simulink model "Blinker_31_exp_func_call_final"  (R2020b)
settings: Solver=FixedStepDiscrete  StartTime=0.0  StopTime=10.0  FixedStep=Ts  RelTol=1e-3  EnableMultiTasking=on
PreLoadFcn:
  | Ts = 0.05;
  | Ts_1 = 0.05;   % for runnable blink_signal
  | Ts_2 = 1;       % for runnable validate_ignition
  | 
  | SetEnumTypeBlink;
undefined symbols (not defined in the file or in its folder): BlinkerValues
libraries: simulink x1
settings Model: SimSIMDOptimization=Portable  Creator=urempel  LastModifiedBy=bnewman
settings DataIOCC: LimitDataPoints=on  SaveFormat=Array  ReturnWorkspaceOutputs=off
settings OptimizationCC: ZeroExternalMemoryAtStartup=off  ZeroInternalMemoryAtStartup=off  LifeSpan=1  EfficientTunableParamExpr=on
settings DebuggingCC: SolverPrmCheckMsg=warning  AllowSymbolicDim=off  SFUnexpectedBacktrackingDiag=warning  SFNoUnconditionalDefaultTransitionDiag=warning  SFExecutionAtInitializationDiag=none  ArithmeticOperatorsInVariantConditions=warning
settings ModelReferenceCC: ModelReferenceNumInstancesAllowed=Single  PropagateSignalLabelsOutOfModel=off
settings SFSimCC: SimUseLocalCustomCode=off  SimGenImportedTypeDefs=on  MATLABDynamicMemAlloc=off  CustomCodeUndefinedFunction=UseInterfaceOnly
settings RTWCC: Description=AUTOSAR  SystemTargetFile=autosar.tlc  GenCodeOnly=on  TemplateMakefile=ert_default_tmf  RTWUseLocalCustomCode=off  IncludeHyperlinkInReport=on  GenerateCodeMetricsReport=on
settings CodeAppCC: IgnoreCustomStorageClasses=off  StateflowObjectComments=on
settings STFCustomTargetCC: ParMdlRefBuildCompliant=on  CompOptLevelCompliant=on  ConcurrentExecutionCompliant=off  IncludeMdlTerminateFcn=off  CombineOutputUpdateFcns=on  SuppressErrorStatus=on  ERTCustomFileBanners=on  SupportNonFinite=off  SupportComplex=off  SupportContinuousTime=off  SupportNonInlinedSFcns=off  RemoveResetFunc=on  MATLABClassNameForMDSCustomization=Simulink.SoftwareTarget.ERTCustomization  CPPClassGenCompliant=off  AutosarCompliant=on  GRTInterface=off  UseToolchainInfoCompliant=on  LookupTableObjectStructAxisOrder=2,1,3,4,...  LUTObjectStructOrderEvenSpacing=Size,Table,Breakpoints  SystemTargetFile=autosar.tlc
settings ERTTargetCC: MultiwordLength=2048  ConcurrentExecutionCompliant=off  IncludeMdlTerminateFcn=off  SuppressErrorStatus=on  SupportNonFinite=off  SupportComplex=off  ModelStepFunctionPrototypeControlCompliant=off  CPPClassGenCompliant=off  AutosarCompliant=on  LookupTableObjectStructAxisOrder=2,1,3,4,...  LUTObjectStructOrderEvenSpacing=Size,Table,Breakpoints  ERTCustomFileTemplate=example_file_process.tlc  ERTFilePackagingFormat=CompactWithDataFile  ConvertIfToSwitch=off  SuppressUnreachableDefaultCases=off
settings ConfigComp: CovMetricSettings=dw  CovSaveCumulativeToWorkspaceVar=on  CovSaveSingleToWorkspaceVar=on  CovExternalEMLEnable=off  CovSFcnEnable=off

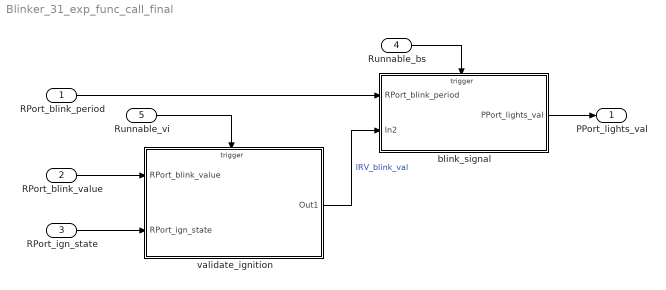
== system Blinker_31_exp_func_call_final ==
  RPort_blink_period : Inport  OutDataTypeStr=uint32
      settings: AttributesFormatString=%<OutDataTypeStr>
  RPort_blink_value : Inport  Port=2  OutDataTypeStr=Enum: BlinkerValues
      settings: AttributesFormatString=%<OutDataTypeStr>
  RPort_ign_state : Inport  Port=3  OutDataTypeStr=boolean
      settings: AttributesFormatString=%<OutDataTypeStr>
  Runnable_bs : Inport  Port=4  SampleTime=Ts_1  OutputFunctionCall=on
  Runnable_vi : Inport  Port=5  SampleTime=Ts_2  OutputFunctionCall=on
  blink_signal : Subsystem
  validate_ignition : Subsystem
  PPort_lights_val : Outport  InitialOutput=0  VectorParamsAs1DForOutWhenUnconnected=off
  wires:
  RPort_blink_value/1 -> validate_ignition/1(RPort_blink_value)
  RPort_ign_state/1 -> validate_ignition/2(RPort_ign_state)
  RPort_blink_period/1 -> blink_signal/1(RPort_blink_period)
  validate_ignition/1(Out1) -> blink_signal/2(In2)  "IRV_blink_val"
  blink_signal/1(PPort_lights_val) -> PPort_lights_val/1
  Runnable_bs/1 -> blink_signal/Trigger
  Runnable_vi/1 -> validate_ignition/Trigger

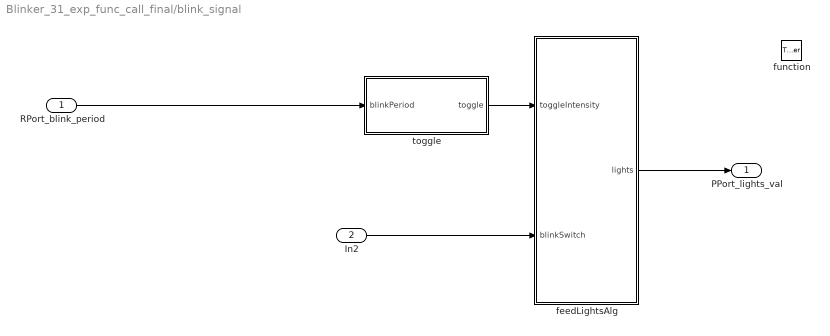
== system Blinker_31_exp_func_call_final/blink_signal ==
  RPort_blink_period : Inport  OutDataTypeStr=uint32
      settings: AttributesFormatString=%<OutDataTypeStr>
  In2 : Inport  Port=2
  function : TriggerPort  TriggerType=function-call  VariantControl=(inherit)  SampleTimeType=periodic  SampleTime=-1
  feedLightsAlg : MATLAB Function  TreatAsAtomicUnit=on
  toggle : Stateflow chart  TreatAsAtomicUnit=on
  PPort_lights_val : Outport  InitialOutput=0  VectorParamsAs1DForOutWhenUnconnected=off
  wires:
  RPort_blink_period/1 -> toggle/1(blinkPeriod)
  feedLightsAlg/1(lights) -> PPort_lights_val/1
  toggle/1(toggle) -> feedLightsAlg/1(toggleIntensity)
  In2/1 -> feedLightsAlg/2(blinkSwitch)

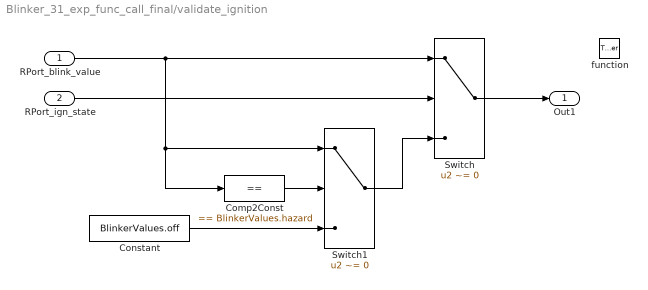
== system Blinker_31_exp_func_call_final/validate_ignition ==
  RPort_blink_value : Inport  OutDataTypeStr=Enum: BlinkerValues
      settings: AttributesFormatString=%<OutDataTypeStr>
  RPort_ign_state : Inport  Port=2  OutDataTypeStr=boolean
      settings: AttributesFormatString=%<OutDataTypeStr>
  function : TriggerPort  TriggerType=function-call  VariantControl=(inherit)  SampleTimeType=periodic  SampleTime=-1
  Comp2Const : simulink/Logic and Bit Operations/Compare To Constant  relop===  const=BlinkerValues.hazard  OutDataTypeStr=boolean
  Constant : Constant  Value=BlinkerValues.off
      settings: AttributesFormatString=%<OutDataTypeStr>
  Switch : Switch  Criteria=u2 ~= 0
  Switch1 : Switch  Criteria=u2 ~= 0
  Out1 : Outport  VectorParamsAs1DForOutWhenUnconnected=off
  wires:
  Switch1/1 -> Switch/3
  RPort_blink_value/1 -> Switch1/1, Comp2Const/1, Switch/1
  Comp2Const/1 -> Switch1/2
  RPort_ign_state/1 -> Switch/2
  Switch/1 -> Out1/1
  Constant/1 -> Switch1/3

== matlab function Blinker_31_exp_func_call_final/blink_signal/feedLightsAlg ==
  data: toggleIntensity input boolean; blinkSwitch input Enum: BlinkerValues; lights output boolean size=[1,2]
function lights = feedLightsAlg(toggleIntensity, blinkSwitch )
%#codegen
switch blinkSwitch
	case BlinkerValues.right
		lights = [false, toggleIntensity];
	case BlinkerValues.left
		lights = [toggleIntensity, false];
	case BlinkerValues.hazard
		lights = [toggleIntensity, toggleIntensity];
	otherwise
		lights = [false, false];
end

== stateflow chart Blinker_31_exp_func_call_final/blink_signal/toggle ==
  (default) -> (junction 2)
  (junction 2) -> (junction 7) [order 1] : [blinkPeriod <= cntr]
  (junction 2) -> (junction 3) [order 2] : {
      | cntr++;
      | }
  (junction 7) -> (junction 8) : {
      | toggle = !toggle;
      | cntr = 1;
      | }
  (junction 8) -> (junction 3)
  data: toggle output boolean =0; blinkPeriod input uint32; cntr local uint32 =0
